simulink model "MotionCore_Phase5B"  (R2026a)
settings: Solver=ode45  StartTime=0  StopTime=1  MaxStep=9.9999999999999995e-07  RelTol=9.9999999999999995e-08  AbsTol=1.0000000000000001e-09
model workspace (MAT data in the model file):
  b.model = 'MotionCore_Phase5B'
  b.Tedge = 1e-06
  b.CPR = 4096
  b.design_max_rpm = 3000
  b.no_load_rpm = 2122.06590789
  b.transition_rate_2000_Hz = 136533.333333
  b.transition_rate_no_load_Hz = 144866.365979
  b.transition_rate_design_Hz = 204800
  b.A_table = [0 0 1 1]
  b.B_table = [0 1 1 0]
  b.delta_table = [0 1 -1 0 -1 0 0 1 1 0 0 -1 0 -1 1 0]
  b.invalid_table = [0 0 0 1 0 0 1 0 0 1 0 0 1 0 0 0]
  b.initial_count = 0
  b.initial_state = 0
  b.test_speeds_rpm = [500 1000 1500 2000]
  b.zoom_start_s = 0.8
  b.zoom_duration_s = 0.0001
  b.compare.copy_atol = 1e-07
  b.compare.copy_rtol = 2e-06
  b.compare.max_true_rpm = 1
  b.compare.max_encoder_rpm = 29.296875
  b.compare.max_current_A = 0.1
  b.compare.max_voltage_V = 0.2
  b.compare.max_duty = 0.0166666666667
  b.compare.max_count = 1
  mc.model = 'MotionCore'
  mc.motor.Ra = 2
  mc.motor.La = 0.002
  mc.motor.Ke = 0.05
  mc.motor.Kt = 0.05
  mc.motor.J = 0.0001
  mc.motor.b = 0.0001
  mc.initial.current_A = 0
  mc.initial.omega_rad_s = 0
  mc.input.step_time_s = 0.05
  mc.input.voltage_before_V = 0
  mc.input.voltage_after_V = 12
  mc.input.load_torque_Nm = 0
  mc.units.rad_s_to_rpm = 9.54929658551
  mc.sim.stop_time_s = 0.8
  mc.sim.solver = 'ode45'
  mc.sim.max_step_s = 5e-05
  mc.sim.rel_tol = 1e-07
  mc.sim.abs_tol = 1e-09
  mc.check.state_relative_tol = 0.0001
  mc.check.steady_relative_tol = 0.002
  mc.check.energy_relative_tol = 0.005
  mc.math.A = [-1000  -25; 500  -1]
  mc.math.B = [500  0; 0  -10000]
  mc.math.C = [1  0; 0  1]
  mc.math.D = [0  0; 0  0]
  mc.math.speed_tf_num = 0.05
  mc.math.speed_tf_den = [2e-07 0.0002002 0.0027]
  mc.math.poles = [-987.32671455; -13.6732854495]
  mc.math.slow_tau_s = 0.0731353121889
  mc.math.electrical_tau_s = 0.001
  mc.math.final_state = [0.444444444444; 222.222222222]
  p3.model = 'MotionCore_Phase3'
  p3.Ts = 0.001
  p3.bandwidth_rad_s = 15
  p3.candidate_bandwidths = [8 15 25]
  p3.test_speeds_rpm = [500 1000 1500 2000]
  p3.step_time_s = 0.05
  p3.stop_time_s = 1
  p3.reference_rpm = 1000
  p3.initial_reference_rpm = 0
  p3.second_step_s = 0.65
  p3.second_step_delta_rpm = 0
  p3.voltage_min_V = 0
  p3.voltage_max_V = 12
  p3.Kd = 0
  p3.derivative_filter_s = 0.005
  p3.antiwindup_time_s = 0.05
  p3.Kb = 20
  p3.integrator_initial_V = 0
  p3.load_Nm = 0
  p3.check.steady_error_rpm = 1
  p3.check.settling_band_fraction = 0.02
  p3.check.settling_limit_s = 0.5
  p3.check.hold_time_s = 0.05
  p3.check.overshoot_limit_pct = 5
  p3.check.reference_relative_tol = 0.0002
  p3.check.identity_relative_tol = 1e-07
  p3.check.energy_relative_tol = 0.005
  p3.A = [-1000  -25; 500  -1]
  p3.B = [500  0; 0  -10000]
  p3.slow_pole_rad_s = 13.6732854495
  p3.fast_pole_rad_s = 987.32671455
  p3.dc_gain_rpm_V = 176.838825658
  p3.Kp = 0.00620355670625
  p3.Ki = 0.0848230016469
  p3.derivative_a = 0.833333333333
  p3.derivative_b = 166.666666667
  p4.model = 'MotionCore_Phase4'
  p4.phase3_model = 'MotionCore_Phase3'
  p4.controller_Ts = 0.001
  p4.Ts = 0.001
  p4.Kp = 0.00620355670625
  p4.Ki = 0.0848230016469
  p4.Kd = 0
  p4.Kb = 20
  p4.fpwm_Hz = 20000
  p4.Tpwm_s = 5e-05
  p4.controller_frequency_Hz = 1000
  p4.Vdc_V = 12
  p4.PWM_BITS = 12
  p4.quantized_duty_experiment = 0
  p4.test_speeds_rpm = [500 1000 1500 2000]
  p4.reference_rpm = 1000
  p4.initial_reference_rpm = 0
  p4.step_time_s = 0.05
  p4.stop_time_s = 1
  p4.load_Nm = 0
  p4.second_step_s = 0.65
  p4.second_step_delta_rpm = 0
  p4.voltage_min_V = 0
  p4.voltage_max_V = 12
  p4.antiwindup_time_s = 0.05
  p4.check.steady_error_rpm = 1
  p4.check.settling_band_fraction = 0.02
  p4.check.settling_limit_s = 0.5
  p4.check.hold_time_s = 0.05
  p4.check.overshoot_limit_pct = 5
  p4.check.reference_relative_tol = 0.0002
  p4.check.identity_relative_tol = 1e-07
  p4.check.energy_relative_tol = 0.005
  p4.check.phase3_regression_relative_tol = 2e-06
  p4.check.pwm_identity_relative_tol = 2e-08
  p4.check.duty_tolerance = 2e-08
  p4.check.max_phase3_regression_abs_rpm = 0.001
  p4.check.max_phase3_regression_abs_current_A = 1e-06
  p5.model = 'MotionCore_Phase5'
  p5.ENCODER_PPR = 1024
  p5.decode_multiplier = 4
  p5.ENCODER_CPR = 4096
  p5.Tenc = 0.001
  p5.theta_initial_rad = 0
  p5.rpm_per_count = 14.6484375
  p5.test_speeds_rpm = [500 1000 1500 2000]
  p5.low_speeds_rpm = [50 100 250 500]
  p5.resolution_sweep_ppr = [128 256 1024 2048]
  p5.run_optional_experiments = 0
  p5.tail_window_s = 0.2
  p5.check.mean_speed_error_rpm = 1
  p5.check.max_tail_speed_error_rpm = 3
  p5.check.overshoot_pct = 5
  p5.check.settling_limit_s = 0.5
  p5.check.identity_tol = 1e-07
  p5.check.transition_tol = 0.0002
  p5.check.copy_relative_tol = 2e-06
  p5.check.copy_absolute_tol = 1e-07
  p5.check.reference_rpm_tol = 29.296875
values from neighbouring files (symbols this model uses):
  b = blocks{k}    [motioncore_plant_signature.m]    (also in run_motioncore_phase3.m = fread(f,Inf,'*uint8'); run_motioncore_phase4.m = fread(f,Inf,'*uint8'); run_motioncore_phase5.m = fread(f,Inf,'*uint8'))
  mc = struct()    [motioncore_init.m]    (also in run_motioncore_phase3.m = getVariable(mw,'mc'); run_motioncore_phase4.m = getVariable(mw3,'mc'); run_motioncore_phase5.m = getVariable(mw,'mc'))
  p3 = motioncore_phase3_init(mc)    [run_motioncore_phase3.m]    (also in run_motioncore_phase4.m = getVariable(mw3,'p3'); run_motioncore_phase5.m = getVariable(mw,'p3'))
  p4 = motioncore_phase4_init(mc,p3)    [run_motioncore_phase4.m]    (also in run_motioncore_phase5.m = getVariable(mw,'p4'))
  p5 = motioncore_phase5_parameters(p5,p3)    [check_motioncore_phase5.m]    (also in motioncore_phase5_reference.m; run_motioncore_phase5.m = motioncore_phase5_parameters(motioncore_phase5_init(p3,p4),p)
settings Model: Creator=peizh  LastModifiedBy=peizh

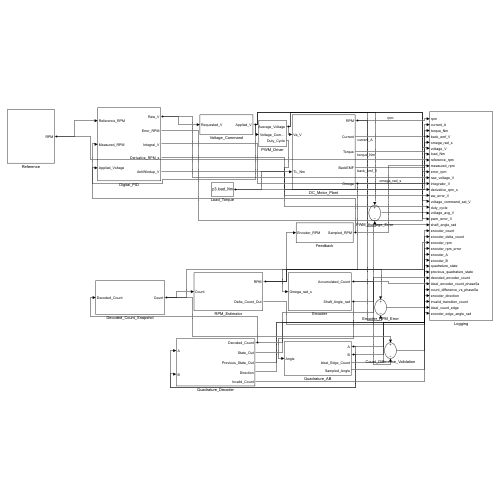
[thumbnail: Simulink's stored preview of the top-level diagram]
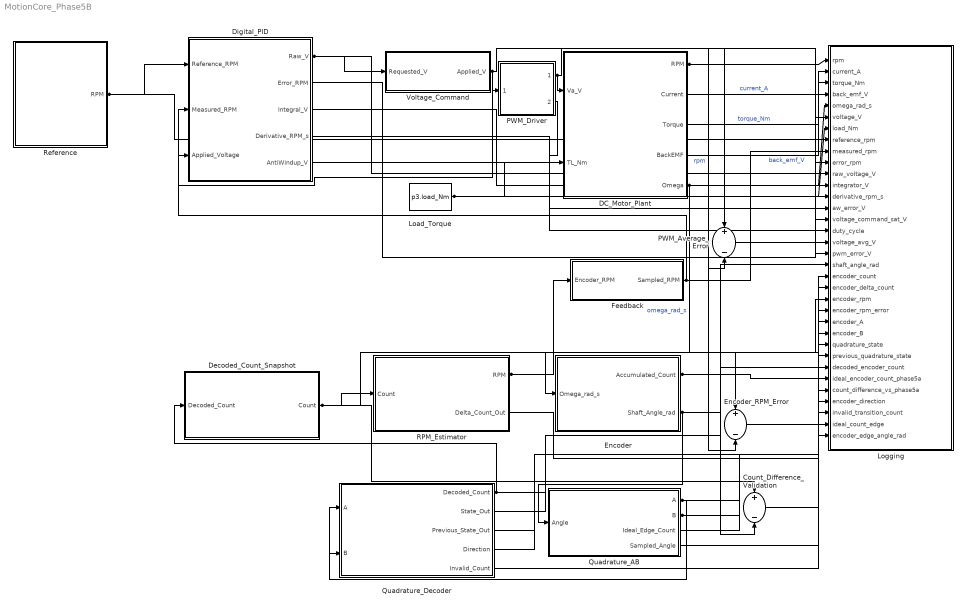
== system MotionCore_Phase5B ==
  Count_Difference_Validation : Sum  Inputs=+-
  DC_Motor_Plant : Subsystem
  Decoded_Count_Snapshot : Subsystem
  Digital_PID : Subsystem
  Encoder : Subsystem
  Encoder_RPM_Error : Sum  Inputs=+-
  Feedback : Subsystem
  Load_Torque : Constant  Value=p3.load_Nm
  Logging : Subsystem
  PWM_Average_Error : Sum  Inputs=+-
  PWM_Driver : Subsystem
  Quadrature_AB : Subsystem
  Quadrature_Decoder : Subsystem
  RPM_Estimator : Subsystem
  Reference : Subsystem
  Voltage_Command : Subsystem
  wires:
  Reference/1(RPM) -> Digital_PID/1(Reference_RPM), Logging/8(reference_rpm)
  Feedback/1(Sampled_RPM) -> Digital_PID/2(Measured_RPM), Logging/9(measured_rpm)
  Digital_PID/1(Raw_V) -> Voltage_Command/1(Requested_V), Logging/11(raw_voltage_V)
  Voltage_Command/1(Applied_V) -> Digital_PID/3(Applied_Voltage), PWM_Driver/1(Voltage_Command_Sat), Logging/6(voltage_V), PWM_Average_Error/2, Logging/15(voltage_command_sat_V)
  PWM_Driver/1(Average_Voltage) -> DC_Motor_Plant/1(Va_V), PWM_Average_Error/1, Logging/17(voltage_avg_V)
  Load_Torque/1 -> DC_Motor_Plant/2(TL_Nm), Logging/7(load_Nm)
  DC_Motor_Plant/1(RPM) -> Logging/1(rpm), Encoder_RPM_Error/2  "rpm"
  DC_Motor_Plant/2(Current) -> Logging/2(current_A)  "current_A"
  DC_Motor_Plant/3(Torque) -> Logging/3(torque_Nm)  "torque_Nm"
  DC_Motor_Plant/4(BackEMF) -> Logging/4(back_emf_V)  "back_emf_V"
  DC_Motor_Plant/5(Omega) -> Logging/5(omega_rad_s), Encoder/1(Omega_rad_s)  "omega_rad_s"
  Digital_PID/2(Error_RPM) -> Logging/10(error_rpm)
  Digital_PID/3(Integral_V) -> Logging/12(integrator_V)
  Digital_PID/4(Derivative_RPM_s) -> Logging/13(derivative_rpm_s)
  Digital_PID/5(AntiWindup_V) -> Logging/14(aw_error_V)
  PWM_Driver/2(Duty_Cycle) -> Logging/16(duty_cycle)
  PWM_Average_Error/1 -> Logging/18(pwm_error_V)
  RPM_Estimator/1(RPM) -> Feedback/1(Encoder_RPM), Encoder_RPM_Error/1, Logging/22(encoder_rpm)
  Encoder/2(Shaft_Angle_rad) -> Logging/19(shaft_angle_rad), Quadrature_AB/1(Angle)
  RPM_Estimator/2(Delta_Count_Out) -> Logging/21(encoder_delta_count)
  Encoder_RPM_Error/1 -> Logging/23(encoder_rpm_error)
  Quadrature_AB/1(A) -> Quadrature_Decoder/1(A), Logging/24(encoder_A)
  Quadrature_AB/2(B) -> Quadrature_Decoder/2(B), Logging/25(encoder_B)
  Quadrature_Decoder/1(Decoded_Count) -> Decoded_Count_Snapshot/1(Decoded_Count), Logging/28(decoded_encoder_count)
  Decoded_Count_Snapshot/1(Count) -> RPM_Estimator/1(Count), Logging/20(encoder_count), Count_Difference_Validation/1
  Encoder/1(Accumulated_Count) -> Count_Difference_Validation/2, Logging/29(ideal_encoder_count_phase5a)
  Quadrature_Decoder/2(State_Out) -> Logging/26(quadrature_state)
  Quadrature_Decoder/3(Previous_State_Out) -> Logging/27(previous_quadrature_state)
  Count_Difference_Validation/1 -> Logging/30(count_difference_vs_phase5a)
  Quadrature_Decoder/4(Direction) -> Logging/31(encoder_direction)
  Quadrature_Decoder/5(Invalid_Count) -> Logging/32(invalid_transition_count)
  Quadrature_AB/3(Ideal_Edge_Count) -> Logging/33(ideal_count_edge)
  Quadrature_AB/4(Sampled_Angle) -> Logging/34(encoder_edge_angle_rad)

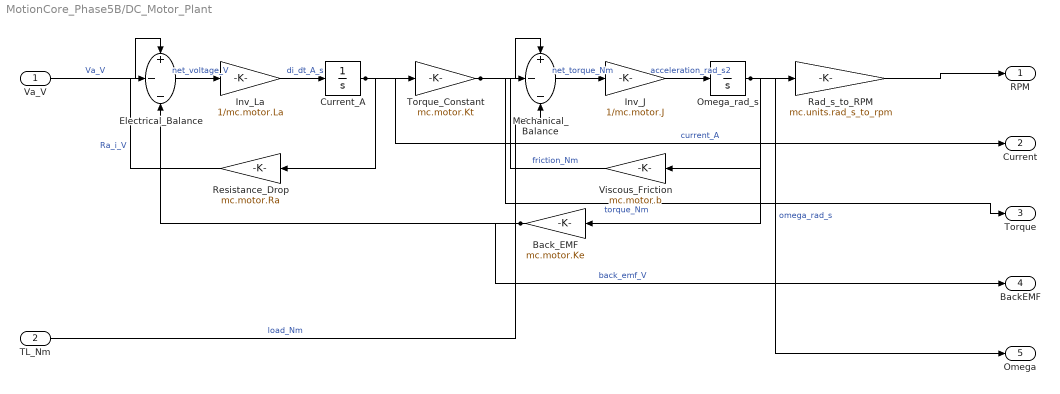
== system MotionCore_Phase5B/DC_Motor_Plant ==
  Va_V : Inport
  TL_Nm : Inport  Port=2
  Back_EMF : Gain  Gain=mc.motor.Ke
  Current_A : Integrator  InitialCondition=mc.initial.current_A
  Electrical_Balance : Sum  Inputs=+--
  Inv_J : Gain  Gain=1/mc.motor.J
  Inv_La : Gain  Gain=1/mc.motor.La
  Mechanical_Balance : Sum  Inputs=+--
  Omega_rad_s : Integrator  InitialCondition=mc.initial.omega_rad_s
  Rad_s_to_RPM : Gain  Gain=mc.units.rad_s_to_rpm
  Resistance_Drop : Gain  Gain=mc.motor.Ra
  Torque_Constant : Gain  Gain=mc.motor.Kt
  Viscous_Friction : Gain  Gain=mc.motor.b
  RPM : Outport
  Current : Outport  Port=2
  Torque : Outport  Port=3
  BackEMF : Outport  Port=4
  Omega : Outport  Port=5
  wires:
  Va_V/1 -> Electrical_Balance/1  "Va_V"
  Electrical_Balance/1 -> Inv_La/1  "net_voltage_V"
  Inv_La/1 -> Current_A/1  "di_dt_A_s"
  Current_A/1 -> Resistance_Drop/1, Torque_Constant/1, Current/1  "current_A"
  Resistance_Drop/1 -> Electrical_Balance/2  "Ra_i_V"
  Torque_Constant/1 -> Mechanical_Balance/1, Torque/1  "torque_Nm"
  Viscous_Friction/1 -> Mechanical_Balance/2  "friction_Nm"
  TL_Nm/1 -> Mechanical_Balance/3  "load_Nm"
  Mechanical_Balance/1 -> Inv_J/1  "net_torque_Nm"
  Inv_J/1 -> Omega_rad_s/1  "acceleration_rad_s2"
  Omega_rad_s/1 -> Viscous_Friction/1, Back_EMF/1, Rad_s_to_RPM/1, Omega/1  "omega_rad_s"
  Back_EMF/1 -> Electrical_Balance/3, BackEMF/1  "back_emf_V"
  Rad_s_to_RPM/1 -> RPM/1

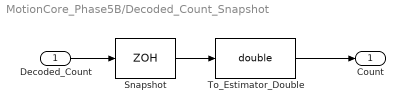
== system MotionCore_Phase5B/Decoded_Count_Snapshot ==
  Decoded_Count : Inport
  Snapshot : ZeroOrderHold  SampleTime=p5.Tenc
  To_Estimator_Double : DataTypeConversion  OutDataTypeStr=double  SaturateOnIntegerOverflow=off  RndMeth=Floor
  Count : Outport
  wires:
  Decoded_Count/1 -> Snapshot/1
  Snapshot/1 -> To_Estimator_Double/1
  To_Estimator_Double/1 -> Count/1

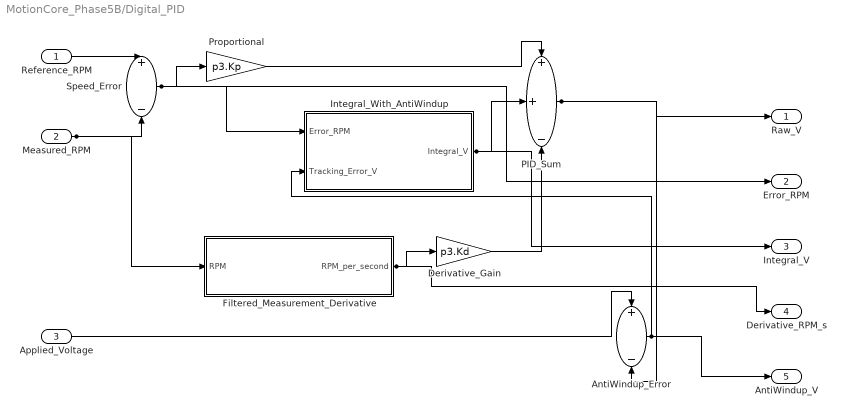
== system MotionCore_Phase5B/Digital_PID ==
  Reference_RPM : Inport
  Measured_RPM : Inport  Port=2
  Applied_Voltage : Inport  Port=3
  AntiWindup_Error : Sum  Inputs=+-
  Derivative_Gain : Gain  Gain=p3.Kd
  Filtered_Measurement_Derivative : Subsystem
  Integral_With_AntiWindup : Subsystem
  PID_Sum : Sum  Inputs=++-
  Proportional : Gain  Gain=p3.Kp
  Speed_Error : Sum  Inputs=+-
  Raw_V : Outport
  Error_RPM : Outport  Port=2
  Integral_V : Outport  Port=3
  Derivative_RPM_s : Outport  Port=4
  AntiWindup_V : Outport  Port=5
  wires:
  Derivative_Gain/1 -> PID_Sum/3
  Filtered_Measurement_Derivative/1(RPM_per_second) -> Derivative_RPM_s/1, Derivative_Gain/1
  Integral_With_AntiWindup/1(Integral_V) -> Integral_V/1, PID_Sum/2
  AntiWindup_Error/1 -> AntiWindup_V/1, Integral_With_AntiWindup/2(Tracking_Error_V)
  PID_Sum/1 -> Raw_V/1, AntiWindup_Error/2
  Applied_Voltage/1 -> AntiWindup_Error/1
  Proportional/1 -> PID_Sum/1
  Speed_Error/1 -> Error_RPM/1, Integral_With_AntiWindup/1(Error_RPM), Proportional/1
  Measured_RPM/1 -> Filtered_Measurement_Derivative/1(RPM), Speed_Error/2
  Reference_RPM/1 -> Speed_Error/1

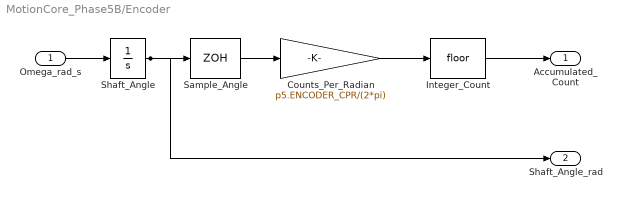
== system MotionCore_Phase5B/Encoder ==
  Omega_rad_s : Inport
  Counts_Per_Radian : Gain  Gain=p5.ENCODER_CPR/(2*pi)
  Integer_Count : Rounding
  Sample_Angle : ZeroOrderHold  SampleTime=p5.Tenc
  Shaft_Angle : Integrator  InitialCondition=p5.theta_initial_rad
  Accumulated_Count : Outport
  Shaft_Angle_rad : Outport  Port=2
  wires:
  Omega_rad_s/1 -> Shaft_Angle/1
  Shaft_Angle/1 -> Sample_Angle/1, Shaft_Angle_rad/1
  Sample_Angle/1 -> Counts_Per_Radian/1
  Counts_Per_Radian/1 -> Integer_Count/1
  Integer_Count/1 -> Accumulated_Count/1

== system MotionCore_Phase5B/Feedback ==
  Encoder_RPM : Inport
  Sample_Speed : ZeroOrderHold  SampleTime=p3.Ts
  Sampled_RPM : Outport
  wires:
  Sample_Speed/1 -> Sampled_RPM/1
  Encoder_RPM/1 -> Sample_Speed/1

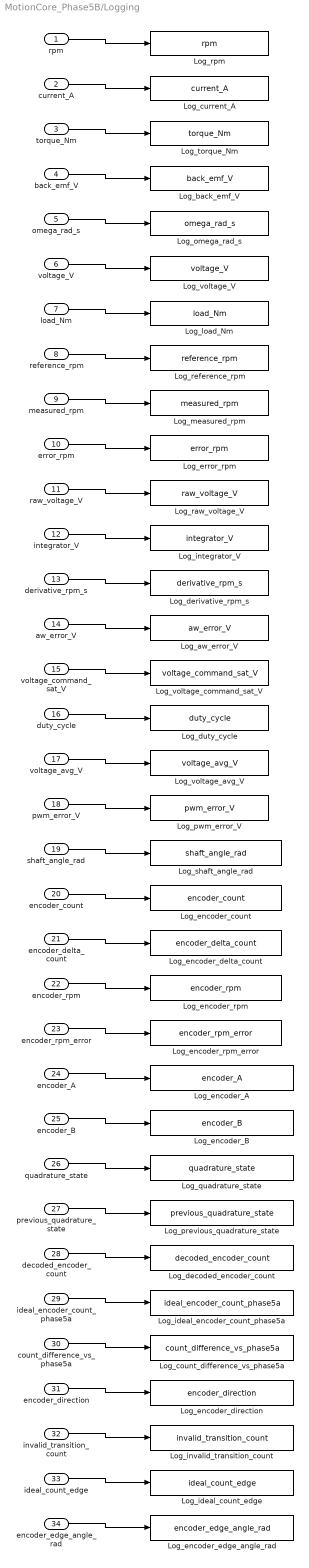
== system MotionCore_Phase5B/Logging ==
  rpm : Inport
  current_A : Inport  Port=2
  torque_Nm : Inport  Port=3
  back_emf_V : Inport  Port=4
  omega_rad_s : Inport  Port=5
  voltage_V : Inport  Port=6
  load_Nm : Inport  Port=7
  reference_rpm : Inport  Port=8
  measured_rpm : Inport  Port=9
  error_rpm : Inport  Port=10
  raw_voltage_V : Inport  Port=11
  integrator_V : Inport  Port=12
  derivative_rpm_s : Inport  Port=13
  aw_error_V : Inport  Port=14
  voltage_command_sat_V : Inport  Port=15
  duty_cycle : Inport  Port=16
  voltage_avg_V : Inport  Port=17
  pwm_error_V : Inport  Port=18
  shaft_angle_rad : Inport  Port=19
  encoder_count : Inport  Port=20
  encoder_delta_count : Inport  Port=21
  encoder_rpm : Inport  Port=22
  encoder_rpm_error : Inport  Port=23
  encoder_A : Inport  Port=24
  encoder_B : Inport  Port=25
  quadrature_state : Inport  Port=26
  previous_quadrature_state : Inport  Port=27
  decoded_encoder_count : Inport  Port=28
  ideal_encoder_count_phase5a : Inport  Port=29
  count_difference_vs_phase5a : Inport  Port=30
  encoder_direction : Inport  Port=31
  invalid_transition_count : Inport  Port=32
  ideal_count_edge : Inport  Port=33
  encoder_edge_angle_rad : Inport  Port=34
  Log_aw_error_V : ToWorkspace  VariableName=aw_error_V  SaveFormat=Timeseries  SampleTime=-1
  Log_back_emf_V : ToWorkspace  VariableName=back_emf_V  SaveFormat=Timeseries  SampleTime=-1
  Log_count_difference_vs_phase5a : ToWorkspace  VariableName=count_difference_vs_phase5a  SaveFormat=Timeseries  SampleTime=-1
  Log_current_A : ToWorkspace  VariableName=current_A  SaveFormat=Timeseries  SampleTime=-1
  Log_decoded_encoder_count : ToWorkspace  VariableName=decoded_encoder_count  SaveFormat=Timeseries  SampleTime=-1
  Log_derivative_rpm_s : ToWorkspace  VariableName=derivative_rpm_s  SaveFormat=Timeseries  SampleTime=-1
  Log_duty_cycle : ToWorkspace  VariableName=duty_cycle  SaveFormat=Timeseries  SampleTime=-1
  Log_encoder_A : ToWorkspace  VariableName=encoder_A  SaveFormat=Timeseries  SampleTime=-1
  Log_encoder_B : ToWorkspace  VariableName=encoder_B  SaveFormat=Timeseries  SampleTime=-1
  Log_encoder_count : ToWorkspace  VariableName=encoder_count  SaveFormat=Timeseries  SampleTime=-1
  Log_encoder_delta_count : ToWorkspace  VariableName=encoder_delta_count  SaveFormat=Timeseries  SampleTime=-1
  Log_encoder_direction : ToWorkspace  VariableName=encoder_direction  SaveFormat=Timeseries  SampleTime=-1
  Log_encoder_edge_angle_rad : ToWorkspace  VariableName=encoder_edge_angle_rad  SaveFormat=Timeseries  SampleTime=-1
  Log_encoder_rpm : ToWorkspace  VariableName=encoder_rpm  SaveFormat=Timeseries  SampleTime=-1
  Log_encoder_rpm_error : ToWorkspace  VariableName=encoder_rpm_error  SaveFormat=Timeseries  SampleTime=-1
  Log_error_rpm : ToWorkspace  VariableName=error_rpm  SaveFormat=Timeseries  SampleTime=-1
  Log_ideal_count_edge : ToWorkspace  VariableName=ideal_count_edge  SaveFormat=Timeseries  SampleTime=-1
  Log_ideal_encoder_count_phase5a : ToWorkspace  VariableName=ideal_encoder_count_phase5a  SaveFormat=Timeseries  SampleTime=-1
  Log_integrator_V : ToWorkspace  VariableName=integrator_V  SaveFormat=Timeseries  SampleTime=-1
  Log_invalid_transition_count : ToWorkspace  VariableName=invalid_transition_count  SaveFormat=Timeseries  SampleTime=-1
  Log_load_Nm : ToWorkspace  VariableName=load_Nm  SaveFormat=Timeseries  SampleTime=-1
  Log_measured_rpm : ToWorkspace  VariableName=measured_rpm  SaveFormat=Timeseries  SampleTime=-1
  Log_omega_rad_s : ToWorkspace  VariableName=omega_rad_s  SaveFormat=Timeseries  SampleTime=-1
  Log_previous_quadrature_state : ToWorkspace  VariableName=previous_quadrature_state  SaveFormat=Timeseries  SampleTime=-1
  Log_pwm_error_V : ToWorkspace  VariableName=pwm_error_V  SaveFormat=Timeseries  SampleTime=-1
  Log_quadrature_state : ToWorkspace  VariableName=quadrature_state  SaveFormat=Timeseries  SampleTime=-1
  Log_raw_voltage_V : ToWorkspace  VariableName=raw_voltage_V  SaveFormat=Timeseries  SampleTime=-1
  Log_reference_rpm : ToWorkspace  VariableName=reference_rpm  SaveFormat=Timeseries  SampleTime=-1
  Log_rpm : ToWorkspace  VariableName=rpm  SaveFormat=Timeseries  SampleTime=-1
  Log_shaft_angle_rad : ToWorkspace  VariableName=shaft_angle_rad  SaveFormat=Timeseries  SampleTime=-1
  Log_torque_Nm : ToWorkspace  VariableName=torque_Nm  SaveFormat=Timeseries  SampleTime=-1
  Log_voltage_V : ToWorkspace  VariableName=voltage_V  SaveFormat=Timeseries  SampleTime=-1
  Log_voltage_avg_V : ToWorkspace  VariableName=voltage_avg_V  SaveFormat=Timeseries  SampleTime=-1
  Log_voltage_command_sat_V : ToWorkspace  VariableName=voltage_command_sat_V  SaveFormat=Timeseries  SampleTime=-1
  wires:
  aw_error_V/1 -> Log_aw_error_V/1
  derivative_rpm_s/1 -> Log_derivative_rpm_s/1
  integrator_V/1 -> Log_integrator_V/1
  raw_voltage_V/1 -> Log_raw_voltage_V/1
  error_rpm/1 -> Log_error_rpm/1
  measured_rpm/1 -> Log_measured_rpm/1
  reference_rpm/1 -> Log_reference_rpm/1
  load_Nm/1 -> Log_load_Nm/1
  voltage_V/1 -> Log_voltage_V/1
  omega_rad_s/1 -> Log_omega_rad_s/1
  back_emf_V/1 -> Log_back_emf_V/1
  torque_Nm/1 -> Log_torque_Nm/1
  current_A/1 -> Log_current_A/1
  rpm/1 -> Log_rpm/1
  voltage_command_sat_V/1 -> Log_voltage_command_sat_V/1
  duty_cycle/1 -> Log_duty_cycle/1
  voltage_avg_V/1 -> Log_voltage_avg_V/1
  pwm_error_V/1 -> Log_pwm_error_V/1
  shaft_angle_rad/1 -> Log_shaft_angle_rad/1
  encoder_count/1 -> Log_encoder_count/1
  encoder_delta_count/1 -> Log_encoder_delta_count/1
  encoder_rpm/1 -> Log_encoder_rpm/1
  encoder_rpm_error/1 -> Log_encoder_rpm_error/1
  encoder_A/1 -> Log_encoder_A/1
  encoder_B/1 -> Log_encoder_B/1
  quadrature_state/1 -> Log_quadrature_state/1
  previous_quadrature_state/1 -> Log_previous_quadrature_state/1
  decoded_encoder_count/1 -> Log_decoded_encoder_count/1
  ideal_encoder_count_phase5a/1 -> Log_ideal_encoder_count_phase5a/1
  count_difference_vs_phase5a/1 -> Log_count_difference_vs_phase5a/1
  encoder_direction/1 -> Log_encoder_direction/1
  invalid_transition_count/1 -> Log_invalid_transition_count/1
  ideal_count_edge/1 -> Log_ideal_count_edge/1
  encoder_edge_angle_rad/1 -> Log_encoder_edge_angle_rad/1

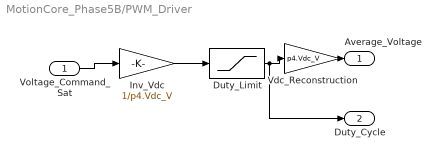
== system MotionCore_Phase5B/PWM_Driver ==
  Voltage_Command_Sat : Inport
  Duty_Limit : Saturate  UpperLimit=1  LowerLimit=0
  Inv_Vdc : Gain  Gain=1/p4.Vdc_V
  Vdc_Reconstruction : Gain  Gain=p4.Vdc_V
  Average_Voltage : Outport
  Duty_Cycle : Outport  Port=2
  wires:
  Voltage_Command_Sat/1 -> Inv_Vdc/1
  Inv_Vdc/1 -> Duty_Limit/1
  Duty_Limit/1 -> Vdc_Reconstruction/1, Duty_Cycle/1
  Vdc_Reconstruction/1 -> Average_Voltage/1

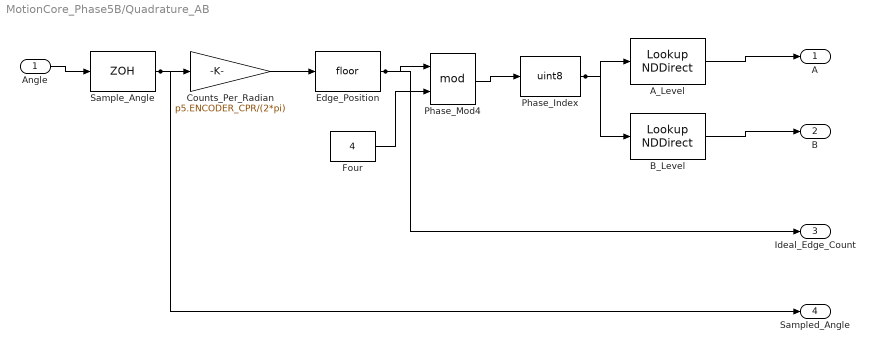
== system MotionCore_Phase5B/Quadrature_AB ==
  Angle : Inport
  A_Level : LookupNDDirect  NumberOfTableDimensions=1  Table=b.A_table
  B_Level : LookupNDDirect  NumberOfTableDimensions=1  Table=b.B_table
  Counts_Per_Radian : Gain  Gain=p5.ENCODER_CPR/(2*pi)
  Edge_Position : Rounding
  Four : Constant  Value=4
  Phase_Index : DataTypeConversion  OutDataTypeStr=uint8  SaturateOnIntegerOverflow=off  RndMeth=Floor
  Phase_Mod4 : Math  Operator=mod
  Sample_Angle : ZeroOrderHold  SampleTime=b.Tedge
  A : Outport
  B : Outport  Port=2
  Ideal_Edge_Count : Outport  Port=3
  Sampled_Angle : Outport  Port=4
  wires:
  Angle/1 -> Sample_Angle/1
  Sample_Angle/1 -> Counts_Per_Radian/1, Sampled_Angle/1
  Counts_Per_Radian/1 -> Edge_Position/1
  Edge_Position/1 -> Phase_Mod4/1, Ideal_Edge_Count/1
  Four/1 -> Phase_Mod4/2
  Phase_Mod4/1 -> Phase_Index/1
  Phase_Index/1 -> A_Level/1, B_Level/1
  A_Level/1 -> A/1
  B_Level/1 -> B/1

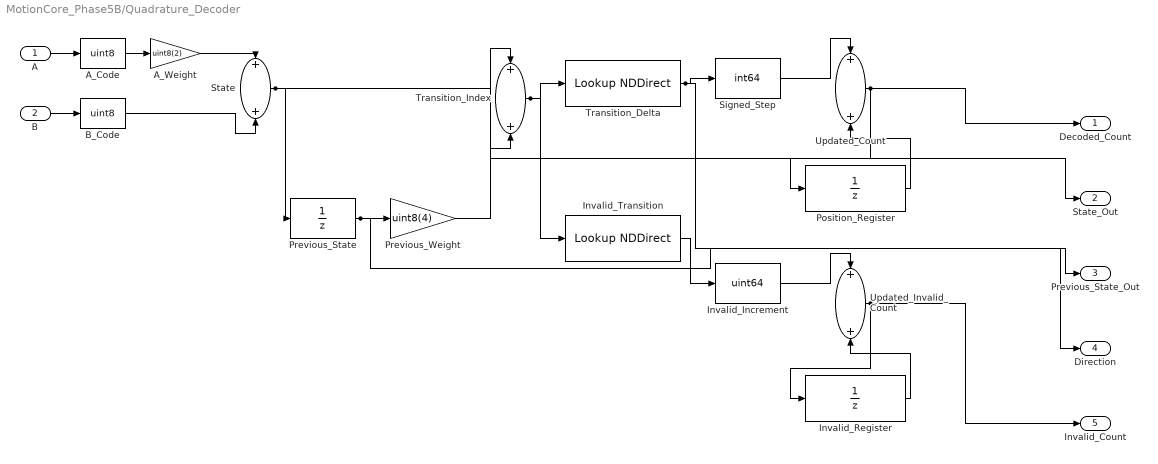
== system MotionCore_Phase5B/Quadrature_Decoder ==
  A : Inport
  B : Inport  Port=2
  A_Code : DataTypeConversion  OutDataTypeStr=uint8  SaturateOnIntegerOverflow=off  RndMeth=Floor
  A_Weight : Gain  Gain=uint8(2)
  B_Code : DataTypeConversion  OutDataTypeStr=uint8  SaturateOnIntegerOverflow=off  RndMeth=Floor
  Invalid_Increment : DataTypeConversion  OutDataTypeStr=uint64  SaturateOnIntegerOverflow=off  RndMeth=Floor
  Invalid_Register : UnitDelay  InitialCondition=uint64(0)  SampleTime=b.Tedge
  Invalid_Transition : LookupNDDirect  NumberOfTableDimensions=1  Table=b.invalid_table
  Position_Register : UnitDelay  InitialCondition=b.initial_count  SampleTime=b.Tedge
  Previous_State : UnitDelay  InitialCondition=b.initial_state  SampleTime=b.Tedge
  Previous_Weight : Gain  Gain=uint8(4)
  Signed_Step : DataTypeConversion  OutDataTypeStr=int64  SaturateOnIntegerOverflow=off  RndMeth=Floor
  State : Sum  OutDataTypeStr=uint8  SaturateOnIntegerOverflow=on
  Transition_Delta : LookupNDDirect  NumberOfTableDimensions=1  Table=b.delta_table
  Transition_Index : Sum  OutDataTypeStr=uint8  SaturateOnIntegerOverflow=on
  Updated_Count : Sum  OutDataTypeStr=int64  SaturateOnIntegerOverflow=on
  Updated_Invalid_Count : Sum  OutDataTypeStr=uint64  SaturateOnIntegerOverflow=on
  Decoded_Count : Outport
  State_Out : Outport  Port=2
  Previous_State_Out : Outport  Port=3
  Direction : Outport  Port=4
  Invalid_Count : Outport  Port=5
  wires:
  A/1 -> A_Code/1
  A_Code/1 -> A_Weight/1
  B/1 -> B_Code/1
  A_Weight/1 -> State/1
  B_Code/1 -> State/2
  State/1 -> Previous_State/1, Transition_Index/2, State_Out/1
  Previous_State/1 -> Previous_Weight/1, Previous_State_Out/1
  Previous_Weight/1 -> Transition_Index/1
  Transition_Index/1 -> Transition_Delta/1, Invalid_Transition/1
  Transition_Delta/1 -> Signed_Step/1, Direction/1
  Signed_Step/1 -> Updated_Count/1
  Position_Register/1 -> Updated_Count/2
  Updated_Count/1 -> Position_Register/1, Decoded_Count/1
  Invalid_Transition/1 -> Invalid_Increment/1
  Invalid_Increment/1 -> Updated_Invalid_Count/1
  Invalid_Register/1 -> Updated_Invalid_Count/2
  Updated_Invalid_Count/1 -> Invalid_Register/1, Invalid_Count/1

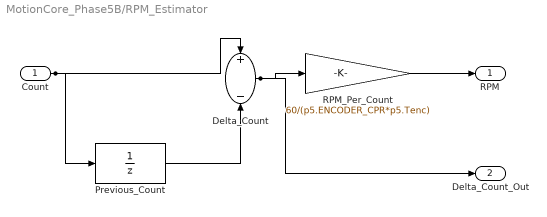
== system MotionCore_Phase5B/RPM_Estimator ==
  Count : Inport
  Delta_Count : Sum  Inputs=+-
  Previous_Count : UnitDelay  InitialCondition=floor(p5.theta_initial_rad*p5.ENCODER_CPR/(2*pi))  SampleTime=p5.Tenc
  RPM_Per_Count : Gain  Gain=60/(p5.ENCODER_CPR*p5.Tenc)
  RPM : Outport
  Delta_Count_Out : Outport  Port=2
  wires:
  Count/1 -> Previous_Count/1, Delta_Count/1
  Previous_Count/1 -> Delta_Count/2
  Delta_Count/1 -> RPM_Per_Count/1, Delta_Count_Out/1
  RPM_Per_Count/1 -> RPM/1

== system MotionCore_Phase5B/Reference ==
  Optional_Second_Change : Step  Time=p3.second_step_s  FinalValue=p3.second_step_delta_rpm  SampleTime=p3.Ts
  Reference_Sum : Sum
  Speed_Request : Step  Time=p3.step_time_s  InitialValue=p3.initial_reference_rpm  FinalValue=p3.reference_rpm  SampleTime=p3.Ts
  RPM : Outport
  wires:
  Reference_Sum/1 -> RPM/1
  Optional_Second_Change/1 -> Reference_Sum/2
  Speed_Request/1 -> Reference_Sum/1

== system MotionCore_Phase5B/Voltage_Command ==
  Requested_V : Inport
  Supply_Limits : Saturate  UpperLimit=p3.voltage_max_V  LowerLimit=p3.voltage_min_V
  Applied_V : Outport
  wires:
  Supply_Limits/1 -> Applied_V/1
  Requested_V/1 -> Supply_Limits/1

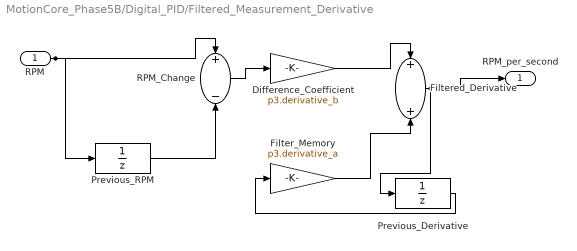
== system MotionCore_Phase5B/Digital_PID/Filtered_Measurement_Derivative ==
  RPM : Inport
  Difference_Coefficient : Gain  Gain=p3.derivative_b
  Filter_Memory : Gain  Gain=p3.derivative_a
  Filtered_Derivative : Sum
  Previous_Derivative : UnitDelay  SampleTime=p3.Ts
  Previous_RPM : UnitDelay  InitialCondition=mc.initial.omega_rad_s*mc.units.rad_s_to_rpm  SampleTime=p3.Ts
  RPM_Change : Sum  Inputs=+-
  RPM_per_second : Outport
  wires:
  Filter_Memory/1 -> Filtered_Derivative/2
  Previous_Derivative/1 -> Filter_Memory/1
  Filtered_Derivative/1 -> RPM_per_second/1, Previous_Derivative/1
  Difference_Coefficient/1 -> Filtered_Derivative/1
  RPM_Change/1 -> Difference_Coefficient/1
  Previous_RPM/1 -> RPM_Change/2
  RPM/1 -> Previous_RPM/1, RPM_Change/1

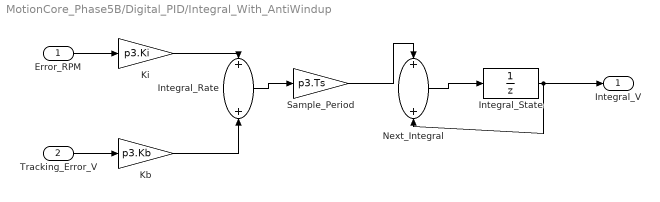
== system MotionCore_Phase5B/Digital_PID/Integral_With_AntiWindup ==
  Error_RPM : Inport
  Tracking_Error_V : Inport  Port=2
  Integral_Rate : Sum
  Integral_State : UnitDelay  InitialCondition=p3.integrator_initial_V  SampleTime=p3.Ts
  Kb : Gain  Gain=p3.Kb
  Ki : Gain  Gain=p3.Ki
  Next_Integral : Sum
  Sample_Period : Gain  Gain=p3.Ts
  Integral_V : Outport
  wires:
  Next_Integral/1 -> Integral_State/1
  Integral_State/1 -> Integral_V/1, Next_Integral/2
  Sample_Period/1 -> Next_Integral/1
  Integral_Rate/1 -> Sample_Period/1
  Kb/1 -> Integral_Rate/2
  Ki/1 -> Integral_Rate/1
  Tracking_Error_V/1 -> Kb/1
  Error_RPM/1 -> Ki/1
